simulink model "PMSM_continous"  (R2019b)
settings: Solver=VariableStepAuto  StartTime=0.0  StopTime=2  FixedStep=1/200000  RelTol=1e-3
model workspace (MAT data in the model file):
  K1 = 5
  K2 = 2000
  Kr = 5
  Ld = 0.01024
  Lq = 0.01024
  P = 10
  Rs = 0.732
  Ts = 5e-05
  Tsim = 5e-05
  Tsim1 = 5e-07
  Udc = 150
  flux = 0.1385
  sigmoid = 0.05
  switch_time = 0.15
undefined symbols (not defined in the file): DiscIntNeverNeededParam, LowerLimit, UpperLimit
libraries: powerlib x9, dspstat3 x4, powerlib_meascontrol x4, simulink x4, fuzblock x4, eeTransforms x2, powerlib_extras x1
settings Model: SimulationMode=accelerator  Creator=Downstream  LastModifiedBy=97252
settings SolverCC: ZeroCrossAlgorithm=Adaptive  AlgebraicLoopSolver=LineSearch
settings DataIOCC: ReturnWorkspaceOutputs=off
settings OptimizationCC: DefaultUnderspecifiedDataType=single  EfficientMapNaN2IntZero=off
settings DebuggingCC: IgnoredZcDiagnostic=none  ArithmeticOperatorsInVariantConditions=warning
settings HardwareCC: TargetBitPerPointer=64  TargetBitPerSizeT=64  TargetBitPerPtrDiffT=64  TargetLongLongMode=on  TargetIntDivRoundTo=Zero  TargetEndianess=LittleEndian  TargetWordSize=64  TargetHWDeviceType=MATLAB Host  ProdEqTarget=off
settings SFSimCC: CustomCodeUndefinedFunction=UseInterfaceOnly
settings CodeAppCC: MaxIdLength=128
settings GRTTargetCC: TargetLangStandard=C89/C90 (ANSI)  CombineOutputUpdateFcns=off  GRTInterface=on

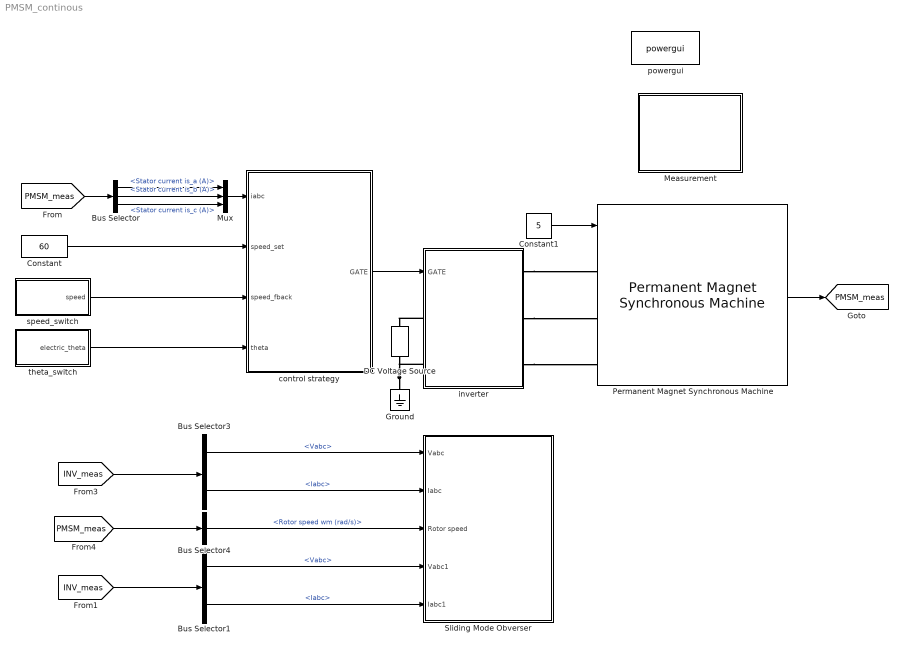
== system PMSM_continous ==
  Bus Selector : BusSelector  OutputSignals=Stator current is_a (A),Stator current is_b (A),Stator current is_c (A)
  Bus Selector1 : BusSelector  OutputSignals=Vabc,Iabc
  Bus Selector3 : BusSelector  OutputSignals=Vabc,Iabc
  Bus Selector4 : BusSelector  OutputSignals=Rotor speed wm (rad/s)
  Constant : Constant  Value=60
  Constant1 : Constant  Value=5
  DC Voltage Source : powerlib/Electrical Sources/DC Voltage Source  Amplitude=Udc  Measurements=None
      settings: SourceProductName=Simscape Electrical
  Ground : powerlib/Elements/Ground  LConnTagsString=a
      settings: SourceProductName=Simscape Electrical
  "Measurement " : Subsystem
  Mux : Mux  Inputs=3
  Permanent Magnet Synchronous Machine : powerlib/Machines/Permanent Magnet Synchronous Machine  NbPhases=3  FluxDistribution=Sinusoidal  RotorType=Salient-pole  MechanicalLoad=Torque Tm  PresetModel=No  ShowDetailedParameters=on  MeasurementBus=off  Resistance=Rs  Inductance=8.5e-3  dqInductances=[Ld, Lq]  La=Ls  MachineConstant=Flux linkage established by magnets (V.s)  Flux=flux  VoltageCst=251.2112  TorqueCst=2.0775  Flat=120  Mechanical=[0.027 0 10 0]  PolePairs=4  InitialConditions=[0,0, 0,0]  InitialConditions5ph=[0 0 0 0 0 0]  RefAngle=Aligned with phase A axis (original Park)  IterativeDiscreteModel=Trapezoidal non iterative  TsBlock=-1  TsPowergui=0
  Sliding Mode Obverser : Subsystem
  control strategy : Subsystem
  "inverter " : Subsystem
  powergui : powerlib/powergui  Priority=1  SimulationMode=Discrete  SampleTime=1/2000000  frequency=60  Iterations=50  frequencyindice=0  Pbase=100e6  ErrMax=1e-4  UnitsV=kV  UnitsW=MW  buscounter=0  FunctionMessages=on  echomessages=on  EnableUseOfTLC=off  CurrentSourceSwitches=off  DisableSnubberDevices=off  DisableRonSwitches=off  DisableVfSwitches=off  DisplayEquations=off  AutomaticDiscreteSolvers=off  SolverType=Tustin/Backward Euler (TBE)  Interpol=off  ExternalGateDelay=off  methode=off  Ts=100  x0status=blocks  SPID=off  SwTol=0  HookPort=off  NonlinearTolerance=1e-4  nMaxIteration=100  ContinueOnMaxIteration=off  RestoreLinks=warning  ResistiveCurrentMeasurement=off  Frange=[0:2:500]  Ylog=off  Xlog=on  ShowGrid=off  save=off  variable=ZData  structure=0  ZoomFFT=off  StartTime=0.0  cycles=1  DisplayStyle=1  fundamental=60  FreqAxis=off  MaxFrequency=1000  frequencyindicesteady=1  RmsSteady=1  display=off
      settings: SourceProductName=Simscape Electrical
  speed_switch : Subsystem
  theta_switch : Subsystem
  tag scope: PMSM_meas=global
  wires:
  Permanent Magnet Synchronous Machine/1 -> [PMSM_meas]
  control strategy/1(GATE) -> "inverter "/1("GATE ")
  [PMSM_meas] -> Bus Selector/1
  Bus Selector/1 -> Mux/1  "<Stator current is_a (A)>"
  Bus Selector/2 -> Mux/2  "<Stator current is_b (A)>"
  Bus Selector/3 -> Mux/3  "<Stator current is_c (A)>"
  Mux/1 -> control strategy/1(iabc)
  Constant1/1 -> Permanent Magnet Synchronous Machine/1
  [PMSM_meas] -> Bus Selector4/1
  Bus Selector4/1 -> Sliding Mode Obverser/3(Rotor speed)  "<Rotor speed wm (rad/s)>"
  Bus Selector3/1 -> Sliding Mode Obverser/1(Vabc)  "<Vabc>"
  Bus Selector3/2 -> Sliding Mode Obverser/2(Iabc)  "<Iabc>"
  [INV_meas] -> Bus Selector3/1
  theta_switch/1(electric_theta) -> control strategy/4(theta)
  speed_switch/1(speed) -> control strategy/3(speed_fback)
  [INV_meas] -> Bus Selector1/1
  Bus Selector1/1 -> Sliding Mode Obverser/4(Vabc1)  "<Vabc>"
  Bus Selector1/2 -> Sliding Mode Obverser/5(Iabc1)  "<Iabc>"
  Constant/1 -> control strategy/2(speed_set)
  connections:
  Ground/LConn1 -- "inverter "/LConn2 -- DC Voltage Source/LConn1
  "inverter "/LConn1 -- DC Voltage Source/RConn1
  "inverter "/RConn1 -- Permanent Magnet Synchronous Machine/LConn1
  "inverter "/RConn2 -- Permanent Magnet Synchronous Machine/LConn2
  "inverter "/RConn3 -- Permanent Magnet Synchronous Machine/LConn3

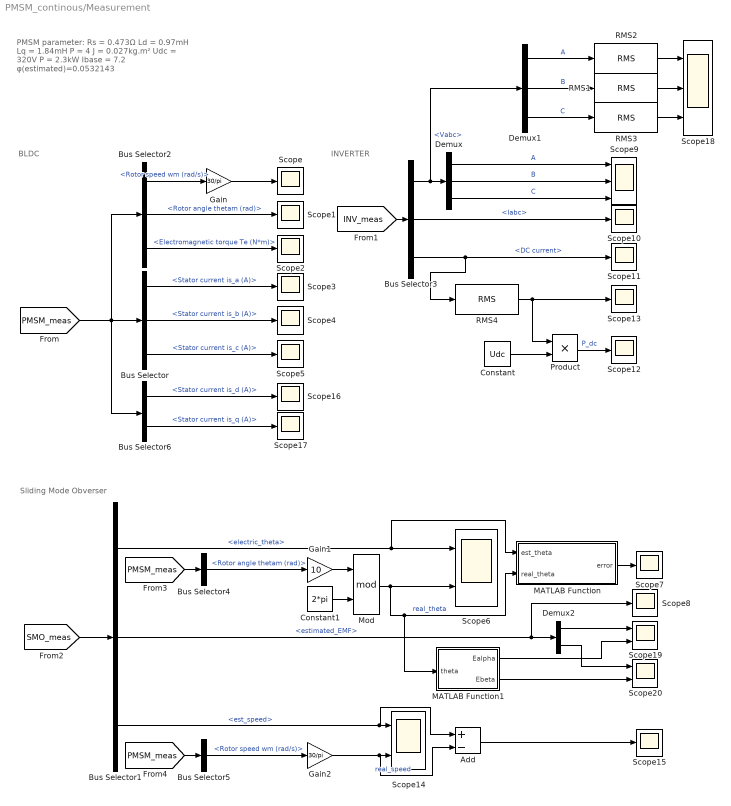
== system PMSM_continous/Measurement  ==
  note: Sliding Mode Obverser
  note: INVERTER
  note: BLDC
  note: PMSM parameter:
      | Rs = 0.473Ω
      | Ld = 0.97mH
      | Lq = 1.84mH
      | P  = 4
      | J   = 0.027kg.m²
      | Udc = 320V
      | P   = 2.3kW
      | Ibase  = 7.2
      | φ(estimated)=0.0532143
  Add : Sum  Inputs=+-
  Bus Selector : BusSelector  OutputSignals=Stator current is_a (A),Stator current is_b (A),Stator current is_c (A)
  Bus Selector1 : BusSelector  OutputSignals=electric_theta,estimated_EMF,est_speed
  Bus Selector2 : BusSelector  OutputSignals=Rotor speed wm (rad/s),Rotor angle thetam (rad),Electromagnetic torque Te (N*m)
  Bus Selector3 : BusSelector  OutputSignals=Vabc,Iabc,DC current
  Bus Selector4 : BusSelector  OutputSignals=Rotor angle thetam (rad)
  Bus Selector5 : BusSelector  OutputSignals=Rotor speed wm (rad/s)
  Bus Selector6 : BusSelector  OutputSignals=Stator current is_d (A),Stator current is_q (A)
  Constant : Constant  Value=Udc
  Constant1 : Constant  Value=2*pi
  Demux : Demux  Outputs=3
  Demux1 : Demux  Outputs=3
  Demux2 : Demux  Outputs=2
  Gain : Gain  Gain=30/pi
  Gain1 : Gain  Gain=10
  Gain2 : Gain  Gain=30/pi
  MATLAB Function : MATLAB Function  TreatAsAtomicUnit=on
  MATLAB Function1 : MATLAB Function  TreatAsAtomicUnit=on
  Mod : Math  Operator=mod  SaturateOnIntegerOverflow=on
  Product : Product
  RMS{1..4} (4 alike) : dspstat3/RMS  run=on  directionMode=Each column  dimension=1  reset_popup=None
  Scope{,1..5,7..8,10..13,15..17} (15 alike) : Scope
  Scope{6,14,19..20} (4 alike) : Scope  NumInputPorts=2
  Scope18 : Scope  NumInputPorts=3
  Scope9 : Scope  NumInputPorts=3
  wires:
  [PMSM_meas] -> Bus Selector6/1, Bus Selector2/1, Bus Selector/1
  Bus Selector2/1 -> Gain/1  "<Rotor speed wm (rad/s)>"
  Bus Selector2/2 -> Scope1/1  "<Rotor angle thetam (rad)>"
  Bus Selector2/3 -> Scope2/1  "<Electromagnetic torque Te (N*m)>"
  Bus Selector/1 -> Scope3/1  "<Stator current is_a (A)>"
  Bus Selector/2 -> Scope4/1  "<Stator current is_b (A)>"
  Bus Selector/3 -> Scope5/1  "<Stator current is_c (A)>"
  [INV_meas] -> Bus Selector3/1
  Bus Selector3/1 -> Demux1/1, Demux/1  "<Vabc>"
  Bus Selector3/2 -> Scope10/1  "<Iabc>"
  Gain/1 -> Scope/1
  Bus Selector3/3 -> RMS4/1, Scope11/1  "<DC current>"
  Constant/1 -> Product/2
  Product/1 -> Scope12/1  "P_dc"
  Demux/2 -> Scope9/2  "B"
  Demux/1 -> Scope9/1  "A"
  Demux/3 -> Scope9/3  "C"
  RMS4/1 -> Product/1, Scope13/1
  [SMO_meas] -> Bus Selector1/1
  Bus Selector1/1 -> MATLAB Function/1(est_theta), Scope6/1  "<electric_theta>"
  Constant1/1 -> Mod/2
  Gain1/1 -> Mod/1
  Bus Selector4/1 -> Gain1/1  "<Rotor angle thetam (rad)>"
  [PMSM_meas] -> Bus Selector4/1
  Mod/1 -> MATLAB Function1/1(theta), MATLAB Function/2(real_theta), Scope6/2  "real_theta"
  MATLAB Function/1(error) -> Scope7/1
  Bus Selector1/3 -> Add/1, Scope14/1  "<est_speed>"
  [PMSM_meas] -> Bus Selector5/1
  Bus Selector5/1 -> Gain2/1  "<Rotor speed wm (rad/s)>"
  Gain2/1 -> Add/2, Scope14/2  "real_speed"
  Add/1 -> Scope15/1
  Bus Selector6/1 -> Scope16/1  "<Stator current is_d (A)>"
  Bus Selector6/2 -> Scope17/1  "<Stator current is_q (A)>"
  Demux1/1 -> RMS2/1  "A"
  Demux1/2 -> RMS1/1  "B"
  Demux1/3 -> RMS3/1  "C"
  RMS2/1 -> Scope18/1
  RMS1/1 -> Scope18/2
  RMS3/1 -> Scope18/3
  Bus Selector1/2 -> Scope8/1, Demux2/1  "<estimated_EMF>"
  Demux2/1 -> Scope19/1
  MATLAB Function1/1(Ealpha) -> Scope19/2
  MATLAB Function1/2(Ebeta) -> Scope20/2
  Demux2/2 -> Scope20/1

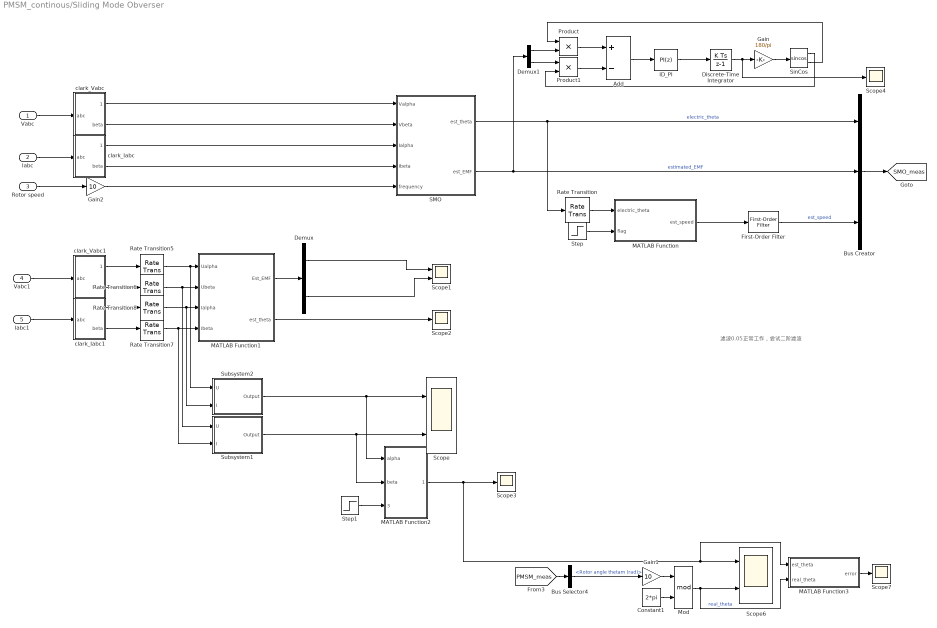
== system PMSM_continous/Sliding Mode Obverser ==
  note: 滤波0.05正常工作，尝试二阶滤波
  Vabc : Inport
  Iabc : Inport  Port=2
  Rotor speed : Inport  Port=3
  Vabc1 : Inport  Port=4
  Iabc1 : Inport  Port=5
  Add : Sum  Inputs=+-
  Bus Creator : BusCreator  Inputs=3
  Bus Selector4 : BusSelector  OutputSignals=Rotor angle thetam (rad)
  Constant1 : Constant  Value=2*pi
  Demux : Demux  Outputs=2
  Demux1 : Demux  Outputs=2
  Discrete-Time Integrator : DiscreteIntegrator  SampleTime=-1  ICPrevOutput=DiscIntNeverNeededParam  ICPrevScaledInput=DiscIntNeverNeededParam
  First-Order Filter : powerlib_meascontrol/Filters/First-Order Filter  FilterType=Lowpass  Tc=1/100  Ts=1/20000  Initialize=off  Vac_Init=[0, 0, 60]  Vdc_Init=0  PlotResponse=off  FreqRange="[0,  200,  1]"
      settings: SourceProductName=Simscape Electrical
  Gain : Gain  Gain=180/pi
  Gain1 : Gain  Gain=10
  Gain2 : Gain  Gain=10
  "ID_PI " : simulink/Continuous/PID Controller  Controller=PI  Form=Parallel  TimeDomain=Discrete-time  SampleTime=-1  IntegratorMethod=Forward Euler  FilterMethod=Forward Euler  ControllerParametersSource=internal  P=300  I=1  D=0  UseFilter=on  N=100  TunerSelectOption=Transfer Function Based (PID Tuner App)  InitialConditionSource=internal  InitialConditionForIntegrator=0  InitialConditionForFilter=0  DifferentiatorICPrevScaledInput=0  ExternalReset=none  TrackingMode=off  Kt=1  LimitOutput=on  UpperSaturationLimit=sqrt(3)/2  LowerSaturationLimit=-sqrt(3)/2  LinearizeAsGain=on  AntiWindupMode=none  Kb=1  POutMin=[]  POutMax=[]  IOutMin=[]  IOutMax=[]  DOutMin=[]  DOutMax=[]  NOutMin=[]  NOutMax=[]  SumOutMin=[]  SumOutMax=[]  SaturationOutMin=[]  SaturationOutMax=[]  PParamMin=[]  PParamMax=[]  IParamMin=[]  IParamMax=[]  DParamMin=[]  DParamMax=[]  NParamMin=[]  NParamMax=[]  KbParamMin=[]  KbParamMax=[]  KtParamMin=[]  KtParamMax=[]  KbOutMin=[]  KbOutMax=[]  KtOutMin=[]  KtOutMax=[]  IntegratorOutMin=[]  IntegratorOutMax=[]  FilterOutMin=[]  FilterOutMax=[]  SumI1OutMin=[]  SumI1OutMax=[]  SumI2OutMin=[]  SumI2OutMax=[]  SumI3OutMin=[]  SumI3OutMax=[]  SumI4OutMin=[]  SumI4OutMax=[]  SumDOutMin=[]  SumDOutMax=[]  DifferentiatorOutMin=[]  DifferentiatorOutMax=[]  FilterDiffOutCoefMin=[]  FilterDiffOutCoefMax=[]  ReciprocalOutMin=[]  ReciprocalOutMax=[]  SumDenOutMin=[]  SumDenOutMax=[]  SumNumOutMin=[]  SumNumOutMax=[]  DivideOutMin=[]  DivideOutMax=[]  IntegratorContinuousStateAttributes=''  IntegratorStateMustResolveToSignalObject=off  IntegratorRTWStateStorageClass=Auto  FilterContinuousStateAttributes=''  FilterStateMustResolveToSignalObject=off  FilterRTWStateStorageClass=Auto  ParallelPVariant=InternalParameters  IdealPVariant=Disabled  IVariant=InternalParameters  DVariant=Disabled  IntegratorVariant=Discrete  SatVariant=Enabled  AWVariant=Passthrough  PCopyVariant=Disabled  TRVariant=Disabled  FdbkBlocksVariant=Forward  IdealPFdbkVariant=Disabled  SatFdbkVariant=Disabled  DerivativeFilterVariant=Disabled  NVariant=Disabled  NCopyVariant=Disabled_SignalSpec  FilterICVariant=Disabled  IntegratorICVariant=InternalICs  ExternalResetVariant=Disabled  TRSumVariant=Passthrough  SumFdbkVariant=Disabled  SumVariant=Sum_PI
  MATLAB Function : MATLAB Function  TreatAsAtomicUnit=on
  MATLAB Function1 : MATLAB Function  TreatAsAtomicUnit=on
  MATLAB Function2 : MATLAB Function  TreatAsAtomicUnit=on
  MATLAB Function3 : MATLAB Function  TreatAsAtomicUnit=on
  Mod : Math  Operator=mod  SaturateOnIntegerOverflow=on
  Product : Product
  Product1 : Product
  Rate Transition : RateTransition  OutPortSampleTime=Ts
  Rate Transition{5..8} (4 alike) : RateTransition  OutPortSampleTime=Tsim
  SMO : MATLAB Function  TreatAsAtomicUnit=on
  Scope : Scope  NumInputPorts=2
  Scope1 : Scope  NumInputPorts=2
  Scope{2..4,7} (4 alike) : Scope
  Scope6 : Scope  NumInputPorts=2
  SinCos : Trigonometry  Operator=sincos
  Step : Step  Time=switch_time/2  SampleTime=Ts
  Step1 : Step  Time=0  After=0  SampleTime=0
  Subsystem1 : Subsystem
  Subsystem2 : Subsystem
  clark_Iabc : Subsystem
  clark_Iabc1 : Subsystem
  clark_Vabc : Subsystem
  clark_Vabc1 : Subsystem
  tag scope: SMO_meas=global
  wires:
  Rate Transition/1 -> MATLAB Function/1(electric_theta)
  MATLAB Function/1(est_speed) -> First-Order Filter/1
  Step/1 -> MATLAB Function/2(flag)
  First-Order Filter/1 -> Bus Creator/3  "est_speed"
  Bus Creator/1 -> [SMO_meas]
  SMO/2(est_EMF) -> Bus Creator/2, Demux1/1  "estimated_EMF"
  SMO/1(est_theta) -> Rate Transition/1, Bus Creator/1  "electric_theta"
  Vabc/1 -> clark_Vabc/1(abc)
  Iabc/1 -> clark_Iabc/1(abc)
  Rotor speed/1 -> Gain2/1
  clark_Vabc1/1(alpha) -> Rate Transition5/1
  clark_Vabc1/2(beta) -> Rate Transition6/1
  clark_Iabc1/1(alpha) -> Rate Transition8/1
  clark_Iabc1/2(beta) -> Rate Transition7/1
  MATLAB Function1/1(Est_EMF) -> Demux/1
  Demux/1 -> Scope1/1
  Demux/2 -> Scope1/2
  MATLAB Function1/2(est_theta) -> Scope2/1
  Iabc1/1 -> clark_Iabc1/1(abc)
  Vabc1/1 -> clark_Vabc1/1(abc)
  [PMSM_meas] -> Bus Selector4/1
  Bus Selector4/1 -> Gain1/1  "<Rotor angle thetam (rad)>"
  Mod/1 -> Scope6/2, MATLAB Function3/2(real_theta)  "real_theta"
  MATLAB Function3/1(error) -> Scope7/1
  Gain1/1 -> Mod/1
  MATLAB Function2/1(Est_theta) -> Scope3/1, MATLAB Function3/1(est_theta), Scope6/1
  Constant1/1 -> Mod/2
  Subsystem2/1(Output) -> Scope/1, MATLAB Function2/1(alpha)
  Subsystem1/1(Output) -> MATLAB Function2/2(beta), Scope/2
  Step1/1 -> MATLAB Function2/3(compansite)
  Rate Transition5/1 -> Subsystem2/1(U), MATLAB Function1/1(Ualpha)
  Rate Transition6/1 -> Subsystem1/1(U), MATLAB Function1/2(Ubeta)
  Rate Transition7/1 -> Subsystem1/2(I), MATLAB Function1/4(Ibeta)
  Rate Transition8/1 -> Subsystem2/2(I), MATLAB Function1/3(Ialpha)
  clark_Iabc/1(alpha) -> SMO/3(Ialpha)
  clark_Vabc/1(alpha) -> SMO/1(Valpha)
  clark_Vabc/2(beta) -> SMO/2(Vbeta)
  clark_Iabc/2(beta) -> SMO/4(Ibeta)
  Gain2/1 -> SMO/5(frequency)
  Demux1/1 -> Product/2
  Demux1/2 -> Product1/1
  Product/1 -> Add/1
  Product1/1 -> Add/2
  Add/1 -> "ID_PI "/1
  "ID_PI "/1 -> Discrete-Time Integrator/1
  Discrete-Time Integrator/1 -> Gain/1, Scope4/1
  SinCos/2 -> Product/1
  SinCos/1 -> Product1/2
  Gain/1 -> SinCos/1

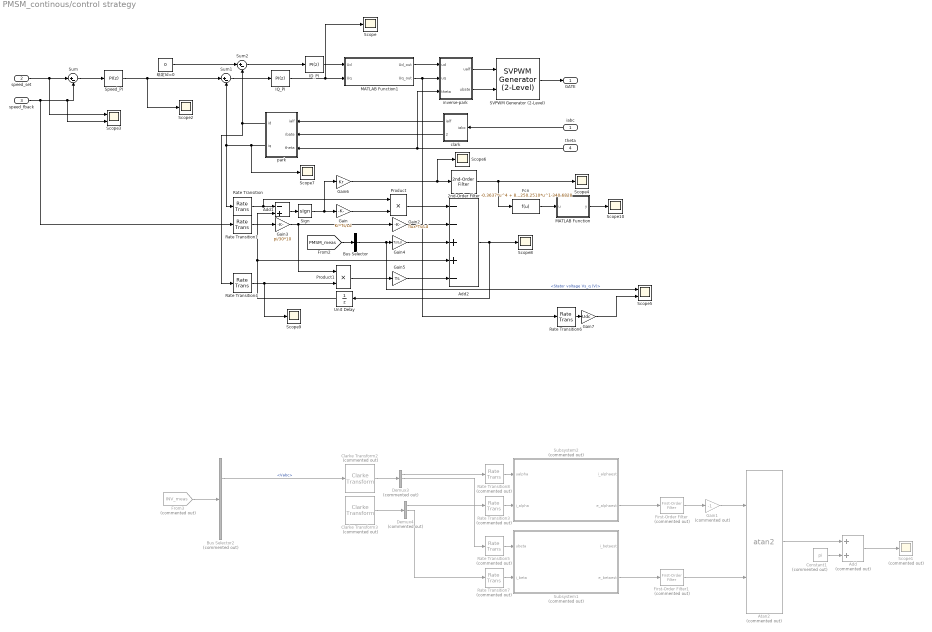
== system PMSM_continous/control strategy ==
  iabc : Inport
  speed_set : Inport  Port=2
  speed_fback : Inport  Port=3
  theta : Inport  Port=4
  2nd-Order Filter : powerlib_extras/Control  Blocks/2nd-Order Filter  FilterType=Lowpass  Fo=50  Zeta=0.707  Initialize=off  Vac_Init=[1 45 60]  Vdc_Init=-0.5  PlotResponse=off  param1=[1 500 1]
      settings: SourceProductName=Simscape Electrical  SourceProductBaseCode=PS
  Add : Sum  Commented=on
  Add1 : Sum  Inputs=-+
  Add2 : Sum  Inputs=--++-
  Atan2 : Trigonometry  Commented=on  Operator=atan2
  Bus Selector : BusSelector  OutputSignals=Stator voltage Vs_q (V)
  Bus Selector2 : BusSelector  Commented=on  OutputSignals=Vabc,Iabc
  Clarke Transform2 : eeTransforms/Clarke Transform  Commented=on  PowerInvariant=off
      settings: SourceProductName=Simscape Electrical  SourceProductBaseCode=PS
  Clarke Transform3 : eeTransforms/Clarke Transform  Commented=on  PowerInvariant=off
      settings: SourceProductName=Simscape Electrical  SourceProductBaseCode=PS
  Constant1 : Constant  Commented=on  Value=pi
  Demux3 : Demux  Commented=on  Outputs=3
  Demux4 : Demux  Commented=on  Outputs=3
  Fcn : Fcn  Expr=-0.3637*u^4 + 8.1652*u^3 - 68.0962*u^2 +250.2510*u^1-340.6828
  First-Order Filter : powerlib_meascontrol/Filters/First-Order Filter  Commented=on  FilterType=Lowpass  Tc=150*pi/30*8*Ts*5  Ts=0  Initialize=off  Vac_Init=[0, 0, 60]  Vdc_Init=0  PlotResponse=off  FreqRange="[0,  200,  1]"
      settings: SourceProductName=Simscape Electrical
  First-Order Filter1 : powerlib_meascontrol/Filters/First-Order Filter  Commented=on  FilterType=Lowpass  Tc=150*pi/30*8*Ts*5  Ts=0  Initialize=off  Vac_Init=[0, 0, 60]  Vdc_Init=0  PlotResponse=off  FreqRange="[0,  200,  1]"
      settings: SourceProductName=Simscape Electrical
  From3 : From  Commented=on  GotoTag=INV_meas  TagVisibility=global
  Gain : Gain  Gain=Kr*Ts/Ld
  Gain1 : Gain  Commented=on  Gain=-1
  Gain2 : Gain  Gain=flux*Ts/Ld
  Gain3 : Gain  Gain=pi/30*10
  Gain4 : Gain  Gain=Ts/Ld
  Gain5 : Gain  Gain=Ts
  Gain6 : Gain  Gain=Kr
  Gain7 : Gain  Gain=Udc
  "ID_PI " : simulink/Continuous/PID Controller  Controller=PI  Form=Parallel  TimeDomain=Discrete-time  SampleTime=Ts  IntegratorMethod=Forward Euler  FilterMethod=Forward Euler  ControllerParametersSource=internal  P=1500*Ld/Udc  I=1500*Rs/Udc  D=0  UseFilter=on  N=100  TunerSelectOption=Transfer Function Based (PID Tuner App)  InitialConditionSource=internal  InitialConditionForIntegrator=0  InitialConditionForFilter=0  DifferentiatorICPrevScaledInput=0  ExternalReset=none  TrackingMode=off  Kt=1  LimitOutput=on  UpperSaturationLimit=sqrt(3)/2  LowerSaturationLimit=-sqrt(3)/2  LinearizeAsGain=on  AntiWindupMode=none  Kb=1  POutMin=[]  POutMax=[]  IOutMin=[]  IOutMax=[]  DOutMin=[]  DOutMax=[]  NOutMin=[]  NOutMax=[]  SumOutMin=[]  SumOutMax=[]  SaturationOutMin=[]  SaturationOutMax=[]  PParamMin=[]  PParamMax=[]  IParamMin=[]  IParamMax=[]  DParamMin=[]  DParamMax=[]  NParamMin=[]  NParamMax=[]  KbParamMin=[]  KbParamMax=[]  KtParamMin=[]  KtParamMax=[]  KbOutMin=[]  KbOutMax=[]  KtOutMin=[]  KtOutMax=[]  IntegratorOutMin=[]  IntegratorOutMax=[]  FilterOutMin=[]  FilterOutMax=[]  SumI1OutMin=[]  SumI1OutMax=[]  SumI2OutMin=[]  SumI2OutMax=[]  SumI3OutMin=[]  SumI3OutMax=[]  SumI4OutMin=[]  SumI4OutMax=[]  SumDOutMin=[]  SumDOutMax=[]  DifferentiatorOutMin=[]  DifferentiatorOutMax=[]  FilterDiffOutCoefMin=[]  FilterDiffOutCoefMax=[]  ReciprocalOutMin=[]  ReciprocalOutMax=[]  SumDenOutMin=[]  SumDenOutMax=[]  SumNumOutMin=[]  SumNumOutMax=[]  DivideOutMin=[]  DivideOutMax=[]  IntegratorContinuousStateAttributes=''  IntegratorStateMustResolveToSignalObject=off  IntegratorRTWStateStorageClass=Auto  FilterContinuousStateAttributes=''  FilterStateMustResolveToSignalObject=off  FilterRTWStateStorageClass=Auto  ParallelPVariant=InternalParameters  IdealPVariant=Disabled  IVariant=InternalParameters  DVariant=Disabled  IntegratorVariant=Discrete  SatVariant=Enabled  AWVariant=Passthrough  PCopyVariant=Disabled  TRVariant=Disabled  FdbkBlocksVariant=Forward  IdealPFdbkVariant=Disabled  SatFdbkVariant=Disabled  DerivativeFilterVariant=Disabled  NVariant=Disabled  NCopyVariant=Disabled_SignalSpec  FilterICVariant=Disabled  IntegratorICVariant=InternalICs  ExternalResetVariant=Disabled  TRSumVariant=Passthrough  SumFdbkVariant=Disabled  SumVariant=Sum_PI
  "IQ_PI " : simulink/Continuous/PID Controller  Controller=PI  Form=Parallel  TimeDomain=Discrete-time  SampleTime=Ts  IntegratorMethod=Forward Euler  FilterMethod=Forward Euler  ControllerParametersSource=internal  P=1500*Ld/Udc  I=1500*Rs/Udc  D=0  UseFilter=on  N=100  TunerSelectOption=Transfer Function Based (PID Tuner App)  InitialConditionSource=internal  InitialConditionForIntegrator=0  InitialConditionForFilter=0  DifferentiatorICPrevScaledInput=0  ExternalReset=none  TrackingMode=off  Kt=1  LimitOutput=on  UpperSaturationLimit=sqrt(3)/2  LowerSaturationLimit=-sqrt(3)/2  LinearizeAsGain=on  AntiWindupMode=none  Kb=1  POutMin=[]  POutMax=[]  IOutMin=[]  IOutMax=[]  DOutMin=[]  DOutMax=[]  NOutMin=[]  NOutMax=[]  SumOutMin=[]  SumOutMax=[]  SaturationOutMin=[]  SaturationOutMax=[]  PParamMin=[]  PParamMax=[]  IParamMin=[]  IParamMax=[]  DParamMin=[]  DParamMax=[]  NParamMin=[]  NParamMax=[]  KbParamMin=[]  KbParamMax=[]  KtParamMin=[]  KtParamMax=[]  KbOutMin=[]  KbOutMax=[]  KtOutMin=[]  KtOutMax=[]  IntegratorOutMin=[]  IntegratorOutMax=[]  FilterOutMin=[]  FilterOutMax=[]  SumI1OutMin=[]  SumI1OutMax=[]  SumI2OutMin=[]  SumI2OutMax=[]  SumI3OutMin=[]  SumI3OutMax=[]  SumI4OutMin=[]  SumI4OutMax=[]  SumDOutMin=[]  SumDOutMax=[]  DifferentiatorOutMin=[]  DifferentiatorOutMax=[]  FilterDiffOutCoefMin=[]  FilterDiffOutCoefMax=[]  ReciprocalOutMin=[]  ReciprocalOutMax=[]  SumDenOutMin=[]  SumDenOutMax=[]  SumNumOutMin=[]  SumNumOutMax=[]  DivideOutMin=[]  DivideOutMax=[]  IntegratorContinuousStateAttributes=''  IntegratorStateMustResolveToSignalObject=off  IntegratorRTWStateStorageClass=Auto  FilterContinuousStateAttributes=''  FilterStateMustResolveToSignalObject=off  FilterRTWStateStorageClass=Auto  ParallelPVariant=InternalParameters  IdealPVariant=Disabled  IVariant=InternalParameters  DVariant=Disabled  IntegratorVariant=Discrete  SatVariant=Enabled  AWVariant=Passthrough  PCopyVariant=Disabled  TRVariant=Disabled  FdbkBlocksVariant=Forward  IdealPFdbkVariant=Disabled  SatFdbkVariant=Disabled  DerivativeFilterVariant=Disabled  NVariant=Disabled  NCopyVariant=Disabled_SignalSpec  FilterICVariant=Disabled  IntegratorICVariant=InternalICs  ExternalResetVariant=Disabled  TRSumVariant=Passthrough  SumFdbkVariant=Disabled  SumVariant=Sum_PI
  MATLAB Function : MATLAB Function  TreatAsAtomicUnit=on
  MATLAB Function1 : MATLAB Function  TreatAsAtomicUnit=on
  Product : Product
  Product1 : Product
  Rate Transition{,1,4,6} (4 alike) : RateTransition  OutPortSampleTime=Ts
  Rate Transition3 : RateTransition  Commented=on  OutPortSampleTime=Ts
  Rate Transition5 : RateTransition  Commented=on  OutPortSampleTime=Ts
  Rate Transition7 : RateTransition  Commented=on  OutPortSampleTime=Ts
  Rate Transition8 : RateTransition  Commented=on  InitialCondition=Ts/10  OutPortSampleTime=Ts
  SVPWM Generator (2-Level) : powerlib_meascontrol/Pulse & Signal Generators/SVPWM Generator (2-Level)  InputType=alpha-beta components  SwitchingPattern=Pattern #1  Fc=20e3  ParUref=[0.8 -30 50]  Ts=0
      settings: SourceProductName=Simscape Electrical  SourceProductBaseCode=PS
  Scope{,2,4,6..10} (8 alike) : Scope
  Scope1 : Scope  Commented=on
  Scope3 : Scope  NumInputPorts=2
  Scope5 : Scope  NumInputPorts=2
  Sign : Signum
  Speed_PI : simulink/Continuous/PID Controller  Controller=PI  Form=Parallel  TimeDomain=Discrete-time  SampleTime=Ts*100  IntegratorMethod=Forward Euler  FilterMethod=Forward Euler  ControllerParametersSource=internal  P=0.05  I=1  D=0  UseFilter=on  N=100  TunerSelectOption=Transfer Function Based (PID Tuner App)  InitialConditionSource=internal  InitialConditionForIntegrator=0  InitialConditionForFilter=0  DifferentiatorICPrevScaledInput=0  ExternalReset=none  TrackingMode=off  Kt=1  LimitOutput=on  UpperSaturationLimit=50  LowerSaturationLimit=-50  LinearizeAsGain=on  AntiWindupMode=none  Kb=1  POutMin=[]  POutMax=[]  IOutMin=[]  IOutMax=[]  DOutMin=[]  DOutMax=[]  NOutMin=[]  NOutMax=[]  SumOutMin=[]  SumOutMax=[]  SaturationOutMin=[]  SaturationOutMax=[]  PParamMin=[]  PParamMax=[]  IParamMin=[]  IParamMax=[]  DParamMin=[]  DParamMax=[]  NParamMin=[]  NParamMax=[]  KbParamMin=[]  KbParamMax=[]  KtParamMin=[]  KtParamMax=[]  KbOutMin=[]  KbOutMax=[]  KtOutMin=[]  KtOutMax=[]  IntegratorOutMin=[]  IntegratorOutMax=[]  FilterOutMin=[]  FilterOutMax=[]  SumI1OutMin=[]  SumI1OutMax=[]  SumI2OutMin=[]  SumI2OutMax=[]  SumI3OutMin=[]  SumI3OutMax=[]  SumI4OutMin=[]  SumI4OutMax=[]  SumDOutMin=[]  SumDOutMax=[]  DifferentiatorOutMin=[]  DifferentiatorOutMax=[]  FilterDiffOutCoefMin=[]  FilterDiffOutCoefMax=[]  ReciprocalOutMin=[]  ReciprocalOutMax=[]  SumDenOutMin=[]  SumDenOutMax=[]  SumNumOutMin=[]  SumNumOutMax=[]  DivideOutMin=[]  DivideOutMax=[]  IntegratorContinuousStateAttributes=''  IntegratorStateMustResolveToSignalObject=off  IntegratorRTWStateStorageClass=Auto  FilterContinuousStateAttributes=''  FilterStateMustResolveToSignalObject=off  FilterRTWStateStorageClass=Auto  ParallelPVariant=InternalParameters  IdealPVariant=Disabled  IVariant=InternalParameters  DVariant=Disabled  IntegratorVariant=Discrete  SatVariant=Enabled  AWVariant=Passthrough  PCopyVariant=Disabled  TRVariant=Disabled  FdbkBlocksVariant=Forward  IdealPFdbkVariant=Disabled  SatFdbkVariant=Disabled  DerivativeFilterVariant=Disabled  NVariant=Disabled  NCopyVariant=Disabled_SignalSpec  FilterICVariant=Disabled  IntegratorICVariant=InternalICs  ExternalResetVariant=Disabled  TRSumVariant=Passthrough  SumFdbkVariant=Disabled  SumVariant=Sum_PI
  Subsystem1 : Subsystem  Commented=on
  Subsystem2 : Subsystem  Commented=on
  Sum : Sum  Inputs=|+-
  Sum1 : Sum  Inputs=|+-
  Sum2 : Sum  Inputs=|+-
  Unit Delay : UnitDelay  SampleTime=-1  HasFrameUpgradeWarning=on
  clark : Subsystem
  inverse-park : Subsystem
  park : Subsystem
  给定Id=0 : Constant  Value=0
  GATE : Outport  VectorParamsAs1DForOutWhenUnconnected=off
  wires:
  SVPWM Generator (2-Level)/1 -> GATE/1
  park/2(iq) -> Scope7/1, Sum1/2, Rate Transition/1
  Sum2/1 -> "ID_PI "/1
  Sum1/1 -> "IQ_PI "/1
  park/1("id ") -> Sum2/2, Rate Transition4/1
  clark/1(ialf) -> park/1(ialf)
  clark/2(ibate) -> park/2(ibate)
  给定Id=0/1 -> Sum2/1
  Sum/1 -> Speed_PI/1
  speed_set/1 -> Scope3/1, Sum/1
  inverse-park/2(ubate) -> SVPWM Generator (2-Level)/2
  inverse-park/1("ualf ") -> SVPWM Generator (2-Level)/1
  Subsystem2/2(e_alphaest) -> First-Order Filter/1
  Subsystem1/2(e_betaest) -> First-Order Filter1/1
  First-Order Filter/1 -> Gain1/1
  Gain1/1 -> Atan2/1
  First-Order Filter1/1 -> Atan2/2
  Atan2/1 -> Add/1
  Constant1/1 -> Add/2
  Demux4/2 -> Rate Transition7/1
  From3/1 -> Bus Selector2/1
  Clarke Transform2/1 -> Demux3/1
  Demux3/1 -> Rate Transition8/1
  Clarke Transform3/1 -> Demux4/1
  Demux3/2 -> Rate Transition5/1
  Demux4/1 -> Rate Transition3/1
  Bus Selector2/1 -> Clarke Transform2/1  "<Vabc>"
  Rate Transition8/1 -> Subsystem2/1(ualpha)
  Rate Transition5/1 -> Subsystem1/1(ubeta)
  Rate Transition3/1 -> Subsystem2/2(i_alpha)
  Rate Transition7/1 -> Subsystem1/2(i_beta)
  Add/1 -> Scope1/1
  iabc/1 -> clark/1(iabc)
  theta/1 -> inverse-park/3(theta), park/3(theta)
  "ID_PI "/1 -> MATLAB Function1/1(Ud)
  "IQ_PI "/1 -> Scope/1, MATLAB Function1/2(Uq)
  MATLAB Function1/1(Ud_out) -> inverse-park/1(ud)
  Speed_PI/1 -> Scope2/1, Sum1/1
  Add1/1 -> Sign/1
  Gain2/1 -> Add2/2
  speed_fback/1 -> Rate Transition1/1, Scope3/2, Sum/2
  Gain3/1 -> Product1/1, Gain2/1
  Gain4/1 -> Add2/3
  Add2/1 -> Scope8/1, Unit Delay/1
  Unit Delay/1 -> Add1/2, Add2/4
  2nd-Order Filter/1 -> Fcn/1, Scope4/1
  Rate Transition/1 -> Product/1, Add1/1
  Rate Transition1/1 -> Gain3/1
  Gain/1 -> Product/2
  Product/1 -> Add2/1
  Rate Transition4/1 -> Product1/2, Scope9/1
  Product1/1 -> Gain5/1
  Gain5/1 -> Add2/5
  Sign/1 -> Gain6/1, Gain/1
  Fcn/1 -> MATLAB Function/1(u)
  MATLAB Function/1(y) -> Scope10/1
  Gain6/1 -> Scope6/1, 2nd-Order Filter/1
  MATLAB Function1/2(Uq_out) -> Rate Transition6/1, inverse-park/2(uq)
  [PMSM_meas] -> Bus Selector/1
  Bus Selector/1 -> Scope5/1, Gain4/1  "<Stator voltage Vs_q (V)>"
  Rate Transition6/1 -> Gain7/1
  Gain7/1 -> Scope5/2

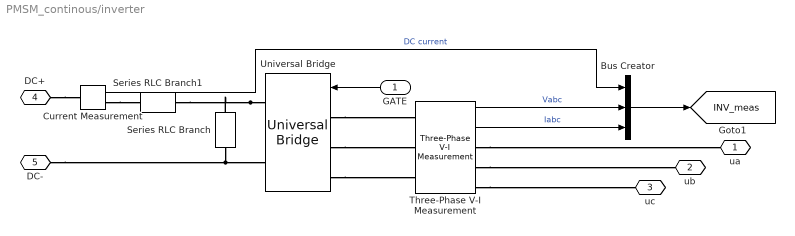
== system PMSM_continous/inverter  ==
  "GATE " : Inport
  Bus Creator : BusCreator  Inputs=3
  Current Measurement : powerlib/Measurements/Current Measurement  PhasorSimulation=off  OutputType=Complex  PSBequivalent=0
      settings: SourceProductName=Simscape Electrical
  Series RLC Branch : powerlib/Elements/Series RLC Branch  LConnTagsString=__new0  RConnTagsString=__new0  BranchType=C  Resistance=1  Inductance=1e-3  SetiL0=off  InitialCurrent=0  Capacitance=5e-3  Setx0=on  InitialVoltage=Udc  Measurements=None
      settings: SourceProductName=Simscape Electrical
  Series RLC Branch1 : powerlib/Elements/Series RLC Branch  LConnTagsString=__new0  RConnTagsString=__new0  BranchType=R  Resistance=0.001  Inductance=1e-3  SetiL0=off  InitialCurrent=0  Capacitance=50e-6  Setx0=off  InitialVoltage=0  Measurements=None
      settings: SourceProductName=Simscape Electrical
  Three-Phase V-I Measurement : powerlib/Measurements/Three-Phase V-I Measurement  VoltageMeasurement=phase-to-ground  SetLabelV=off  LabelV=Vabc  Vpu=off  VpuLL=off  CurrentMeasurement=yes  SetLabelI=off  LabelI=Iabc  Ipu=off  Pbase=100e6  Vbase=500e3  OutputType=Complex  PhasorSimulation=off  PSBequivalent=0
      settings: SourceProductName=Simscape Electrical
  Universal Bridge : powerlib/Power Electronics/Universal Bridge  Arms=3  SnubberResistance=1e5  SnubberCapacitance=inf  Device=IGBT / Diodes  Ron=1e-3  Lon=0  ForwardVoltages="[  0  0  ]"  ForwardVoltage=0  GTOparameters=[ 10e-6 , 20e-6 ]  IGBTparameters=[ 1e-6 , 2e-6 ]  Measurements=None  Measurements_2=None  converterType=Rectifier
      settings: SourceProductName=Simscape Electrical
  ua : PMIOPort  Side=Right
  ub : PMIOPort  Port=2  Side=Right
  uc : PMIOPort  Port=3  Side=Right
  DC+ : PMIOPort  Port=4  Side=Left
  DC- : PMIOPort  Port=5  Side=Left
  tag scope: INV_meas=global
  wires:
  "GATE "/1 -> Universal Bridge/1
  Three-Phase V-I Measurement/1 -> Bus Creator/2  "Vabc"
  Bus Creator/1 -> [INV_meas]
  Three-Phase V-I Measurement/2 -> Bus Creator/3  "Iabc"
  Current Measurement/1 -> Bus Creator/1  "DC current"
  connections:
  Universal Bridge/LConn1 -- Three-Phase V-I Measurement/LConn1
  Universal Bridge/LConn2 -- Three-Phase V-I Measurement/LConn2
  DC-/RConn1 -- Series RLC Branch/RConn1 -- Universal Bridge/RConn2
  Universal Bridge/LConn3 -- Three-Phase V-I Measurement/LConn3
  Three-Phase V-I Measurement/RConn1 -- ua/RConn1
  Three-Phase V-I Measurement/RConn2 -- ub/RConn1
  Three-Phase V-I Measurement/RConn3 -- uc/RConn1
  Universal Bridge/RConn1 -- Series RLC Branch1/RConn1 -- Series RLC Branch/LConn1
  DC+/RConn1 -- Current Measurement/LConn1
  Current Measurement/RConn1 -- Series RLC Branch1/LConn1

== system PMSM_continous/speed_switch ==
  Bus Selector4 : BusSelector  OutputSignals=Rotor speed wm (rad/s)
  Gain : Gain  Gain=30/pi
  speed : Outport  VectorParamsAs1DForOutWhenUnconnected=off
  wires:
  [PMSM_meas] -> Bus Selector4/1
  Bus Selector4/1 -> Gain/1  "<Rotor speed wm (rad/s)>"
  Gain/1 -> speed/1

== system PMSM_continous/theta_switch ==
  Bus Selector4 : BusSelector  OutputSignals=Rotor angle thetam (rad)
  Constant1 : Constant  Value=2*pi
  Gain1 : Gain  Gain=10
  Mod : Math  Operator=mod  SaturateOnIntegerOverflow=on
  electric_theta : Outport  VectorParamsAs1DForOutWhenUnconnected=off
  wires:
  [PMSM_meas] -> Bus Selector4/1
  Bus Selector4/1 -> Gain1/1  "<Rotor angle thetam (rad)>"
  Gain1/1 -> Mod/1
  Constant1/1 -> Mod/2
  Mod/1 -> electric_theta/1  "real_theta"

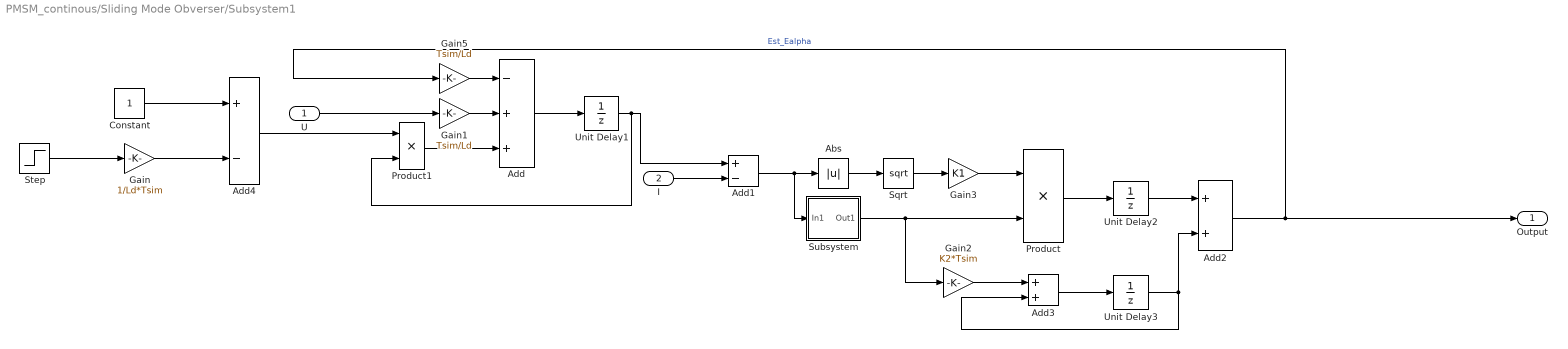
== system PMSM_continous/Sliding Mode Obverser/Subsystem1 ==
  U : Inport
  I : Inport  Port=2
  Abs : Abs
  Add : Sum  Inputs=-++
  Add1 : Sum  Inputs=+-
  Add2 : Sum
  Add3 : Sum
  Add4 : Sum  Inputs=+-
  Constant : Constant  SampleTime=Tsim
  Gain : Gain  Gain=1/Ld*Tsim
  Gain1 : Gain  Gain=Tsim/Ld
  Gain2 : Gain  Gain=K2*Tsim
  Gain3 : Gain  Gain=K1
  Gain5 : Gain  Gain=Tsim/Ld
  Product : Product
  Product1 : Product
  Sqrt : Sqrt  SaturateOnIntegerOverflow=on
  Step : Step  Time=3  Before=0.732  After=0.732+1.3  SampleTime=Tsim
  Subsystem : Subsystem
  Unit Delay1 : UnitDelay  SampleTime=-1  HasFrameUpgradeWarning=on
  Unit Delay2 : UnitDelay  SampleTime=-1  HasFrameUpgradeWarning=on
  Unit Delay3 : UnitDelay  SampleTime=-1  HasFrameUpgradeWarning=on
  Output : Outport
  wires:
  Gain/1 -> Add4/2
  Step/1 -> Gain/1
  Constant/1 -> Add4/1
  Add4/1 -> Product1/1
  Unit Delay3/1 -> Add2/2, Add3/2
  Unit Delay2/1 -> Add2/1
  Unit Delay1/1 -> Product1/2, Add1/1
  Abs/1 -> Sqrt/1
  Add1/1 -> Subsystem/1(In1), Abs/1
  I/1 -> Add1/2
  U/1 -> Gain1/1
  Sqrt/1 -> Gain3/1
  Gain3/1 -> Product/1
  Product1/1 -> Add/3
  Add2/1 -> Gain5/1, Output/1  "Est_Ealpha"
  Gain1/1 -> Add/2
  Subsystem/1(Out1) -> Product/2, Gain2/1
  Product/1 -> Unit Delay2/1
  Gain5/1 -> Add/1
  Add/1 -> Unit Delay1/1
  Add3/1 -> Unit Delay3/1
  Gain2/1 -> Add3/1

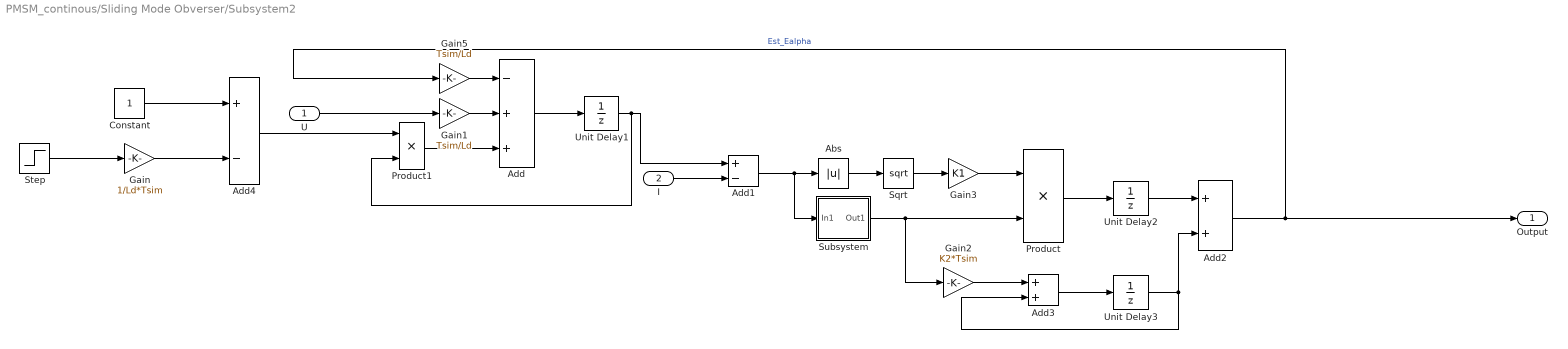
== system PMSM_continous/Sliding Mode Obverser/Subsystem2 ==
  U : Inport
  I : Inport  Port=2
  Abs : Abs
  Add : Sum  Inputs=-++
  Add1 : Sum  Inputs=+-
  Add2 : Sum
  Add3 : Sum
  Add4 : Sum  Inputs=+-
  Constant : Constant  SampleTime=Tsim
  Gain : Gain  Gain=1/Ld*Tsim
  Gain1 : Gain  Gain=Tsim/Ld
  Gain2 : Gain  Gain=K2*Tsim
  Gain3 : Gain  Gain=K1
  Gain5 : Gain  Gain=Tsim/Ld
  Product : Product
  Product1 : Product
  Sqrt : Sqrt  SaturateOnIntegerOverflow=on
  Step : Step  Time=3  Before=0.732  After=0.732+1.3  SampleTime=Tsim
  Subsystem : Subsystem
  Unit Delay1 : UnitDelay  SampleTime=-1  HasFrameUpgradeWarning=on
  Unit Delay2 : UnitDelay  SampleTime=-1  HasFrameUpgradeWarning=on
  Unit Delay3 : UnitDelay  SampleTime=-1  HasFrameUpgradeWarning=on
  Output : Outport
  wires:
  Gain2/1 -> Add3/1
  Add3/1 -> Unit Delay3/1
  Add/1 -> Unit Delay1/1
  Gain5/1 -> Add/1
  Product/1 -> Unit Delay2/1
  Subsystem/1(Out1) -> Gain2/1, Product/2
  Gain1/1 -> Add/2
  Add2/1 -> Output/1, Gain5/1  "Est_Ealpha"
  Product1/1 -> Add/3
  Gain3/1 -> Product/1
  Sqrt/1 -> Gain3/1
  U/1 -> Gain1/1
  I/1 -> Add1/2
  Add1/1 -> Subsystem/1(In1), Abs/1
  Abs/1 -> Sqrt/1
  Unit Delay1/1 -> Add1/1, Product1/2
  Unit Delay2/1 -> Add2/1
  Unit Delay3/1 -> Add3/2, Add2/2
  Add4/1 -> Product1/1
  Constant/1 -> Add4/1
  Step/1 -> Gain/1
  Gain/1 -> Add4/2

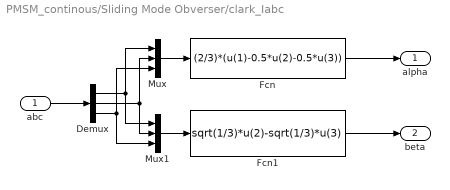
== system PMSM_continous/Sliding Mode Obverser/clark_Iabc ==
  abc : Inport
  Demux : Demux  Outputs=3
  Fcn : Fcn  Expr=(2/3)*(u(1)-0.5*u(2)-0.5*u(3))
  Fcn1 : Fcn  Expr=sqrt(1/3)*u(2)-sqrt(1/3)*u(3)
  Mux : Mux  Inputs=3
  Mux1 : Mux  Inputs=3
  alpha : Outport  VectorParamsAs1DForOutWhenUnconnected=off
  beta : Outport  Port=2  VectorParamsAs1DForOutWhenUnconnected=off
  wires:
  abc/1 -> Demux/1
  Fcn/1 -> alpha/1
  Demux/1 -> Mux1/1, Mux/1
  Demux/2 -> Mux1/2, Mux/2
  Mux/1 -> Fcn/1
  Demux/3 -> Mux1/3, Mux/3
  Fcn1/1 -> beta/1
  Mux1/1 -> Fcn1/1

== system PMSM_continous/Sliding Mode Obverser/clark_Iabc1 ==
  abc : Inport
  Demux : Demux  Outputs=3
  Fcn : Fcn  Expr=(2/3)*(u(1)-0.5*u(2)-0.5*u(3))
  Fcn1 : Fcn  Expr=sqrt(1/3)*u(2)-sqrt(1/3)*u(3)
  Mux : Mux  Inputs=3
  Mux1 : Mux  Inputs=3
  alpha : Outport  VectorParamsAs1DForOutWhenUnconnected=off
  beta : Outport  Port=2  VectorParamsAs1DForOutWhenUnconnected=off
  wires:
  abc/1 -> Demux/1
  Fcn/1 -> alpha/1
  Demux/1 -> Mux1/1, Mux/1
  Demux/2 -> Mux1/2, Mux/2
  Mux/1 -> Fcn/1
  Demux/3 -> Mux1/3, Mux/3
  Fcn1/1 -> beta/1
  Mux1/1 -> Fcn1/1

== system PMSM_continous/Sliding Mode Obverser/clark_Vabc ==
  abc : Inport
  Demux : Demux  Outputs=3
  Fcn : Fcn  Expr=(2/3)*(u(1)-0.5*u(2)-0.5*u(3))
  Fcn1 : Fcn  Expr=sqrt(1/3)*u(2)-sqrt(1/3)*u(3)
  Mux : Mux  Inputs=3
  Mux1 : Mux  Inputs=3
  alpha : Outport  VectorParamsAs1DForOutWhenUnconnected=off
  beta : Outport  Port=2  VectorParamsAs1DForOutWhenUnconnected=off
  wires:
  abc/1 -> Demux/1
  Fcn/1 -> alpha/1
  Demux/1 -> Mux1/1, Mux/1
  Demux/2 -> Mux1/2, Mux/2
  Mux/1 -> Fcn/1
  Demux/3 -> Mux1/3, Mux/3
  Fcn1/1 -> beta/1
  Mux1/1 -> Fcn1/1

== system PMSM_continous/Sliding Mode Obverser/clark_Vabc1 ==
  abc : Inport
  Demux : Demux  Outputs=3
  Fcn : Fcn  Expr=(2/3)*(u(1)-0.5*u(2)-0.5*u(3))
  Fcn1 : Fcn  Expr=sqrt(1/3)*u(2)-sqrt(1/3)*u(3)
  Mux : Mux  Inputs=3
  Mux1 : Mux  Inputs=3
  alpha : Outport  VectorParamsAs1DForOutWhenUnconnected=off
  beta : Outport  Port=2  VectorParamsAs1DForOutWhenUnconnected=off
  wires:
  abc/1 -> Demux/1
  Fcn/1 -> alpha/1
  Demux/1 -> Mux1/1, Mux/1
  Demux/2 -> Mux1/2, Mux/2
  Mux/1 -> Fcn/1
  Demux/3 -> Mux1/3, Mux/3
  Fcn1/1 -> beta/1
  Mux1/1 -> Fcn1/1

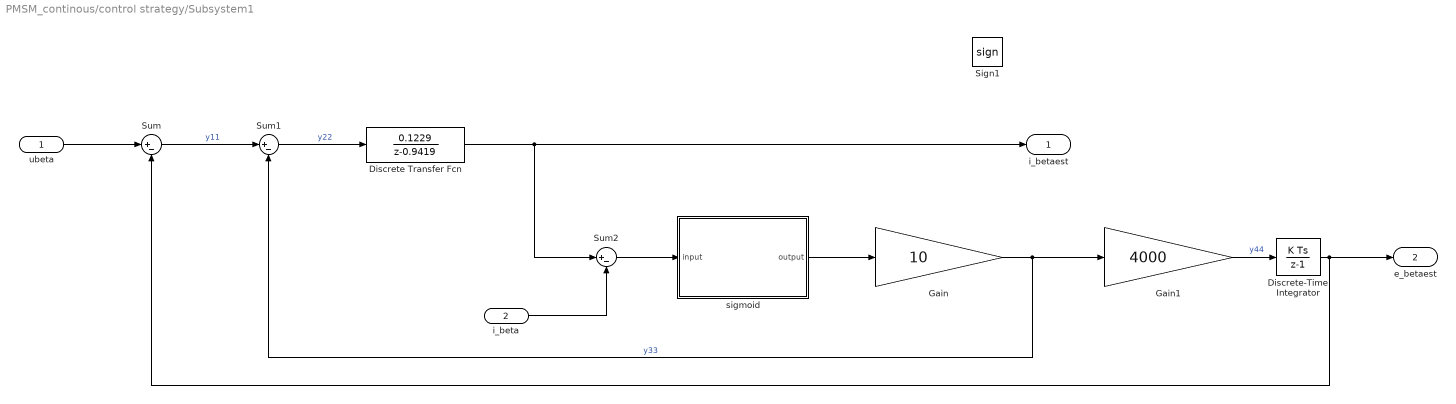
== system PMSM_continous/control strategy/Subsystem1 ==
  ubeta : Inport
  i_beta : Inport  Port=2
  Discrete Transfer Fcn : DiscreteTransferFcn  Numerator=[0.1229]  Denominator=[1 -0.9419]  SampleTime=Ts
  Discrete-Time Integrator : DiscreteIntegrator  SampleTime=Ts  UpperSaturationLimit=UpperLimit  LowerSaturationLimit=LowerLimit  ICPrevOutput=DiscIntNeverNeededParam  ICPrevScaledInput=DiscIntNeverNeededParam
  Gain : Gain  Gain=10
  Gain1 : Gain  Gain=4000
  Sign1 : Signum
  Sum : Sum  Inputs=|+-
  Sum1 : Sum  Inputs=|+-
  Sum2 : Sum  Inputs=|+-
  sigmoid : Subsystem
  i_betaest : Outport  VectorParamsAs1DForOutWhenUnconnected=off
  e_betaest : Outport  Port=2  VectorParamsAs1DForOutWhenUnconnected=off
  wires:
  Sum2/1 -> sigmoid/1(input)
  Gain/1 -> Gain1/1, Sum1/2  "y33"
  i_beta/1 -> Sum2/2
  Discrete Transfer Fcn/1 -> Sum2/1, i_betaest/1
  Sum/1 -> Sum1/1  "y11"
  ubeta/1 -> Sum/1
  Sum1/1 -> Discrete Transfer Fcn/1  "y22"
  Gain1/1 -> Discrete-Time Integrator/1  "y44"
  sigmoid/1(output) -> Gain/1
  Discrete-Time Integrator/1 -> e_betaest/1, Sum/2

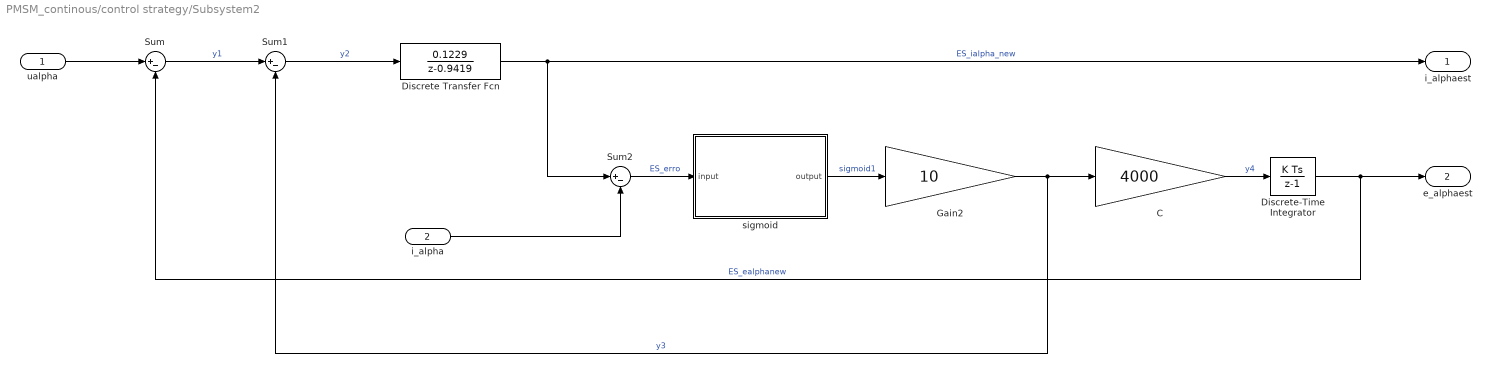
== system PMSM_continous/control strategy/Subsystem2 ==
  ualpha : Inport
  i_alpha : Inport  Port=2
  C : Gain  Gain=4000
  Discrete Transfer Fcn : DiscreteTransferFcn  Numerator=[0.1229]  Denominator=[1 -0.9419]  SampleTime=Ts
  Discrete-Time Integrator : DiscreteIntegrator  SampleTime=Ts  UpperSaturationLimit=UpperLimit  LowerSaturationLimit=LowerLimit  ICPrevOutput=DiscIntNeverNeededParam  ICPrevScaledInput=DiscIntNeverNeededParam
  Gain2 : Gain  Gain=10
  Sum : Sum  Inputs=|+-
  Sum1 : Sum  Inputs=|+-
  Sum2 : Sum  Inputs=|+-
  sigmoid : Subsystem
  i_alphaest : Outport  VectorParamsAs1DForOutWhenUnconnected=off
  e_alphaest : Outport  Port=2  VectorParamsAs1DForOutWhenUnconnected=off
  wires:
  C/1 -> Discrete-Time Integrator/1  "y4"
  Sum1/1 -> Discrete Transfer Fcn/1  "y2"
  ualpha/1 -> Sum/1
  sigmoid/1(output) -> Gain2/1  "sigmoid1"
  Sum/1 -> Sum1/1  "y1"
  Discrete Transfer Fcn/1 -> i_alphaest/1, Sum2/1  "ES_ialpha_new"
  i_alpha/1 -> Sum2/2
  Sum2/1 -> sigmoid/1(input)  "ES_erro"
  Gain2/1 -> C/1, Sum1/2  "y3"
  Discrete-Time Integrator/1 -> Sum/2, e_alphaest/1  "ES_ealphanew"

== system PMSM_continous/control strategy/clark ==
  iabc : Inport
  Demux : Demux  Outputs=3
  Fcn : Fcn  Expr=(2/3)*(u(1)-0.5*u(2)-0.5*u(3))
  Fcn1 : Fcn  Expr=sqrt(1/3)*u(2)-sqrt(1/3)*u(3)
  Mux : Mux  Inputs=3
  Mux1 : Mux  Inputs=3
  ialf : Outport  VectorParamsAs1DForOutWhenUnconnected=off
  ibate : Outport  Port=2  VectorParamsAs1DForOutWhenUnconnected=off
  wires:
  iabc/1 -> Demux/1
  Fcn/1 -> ialf/1
  Demux/1 -> Mux1/1, Mux/1
  Demux/2 -> Mux1/2, Mux/2
  Mux/1 -> Fcn/1
  Demux/3 -> Mux1/3, Mux/3
  Fcn1/1 -> ibate/1
  Mux1/1 -> Fcn1/1

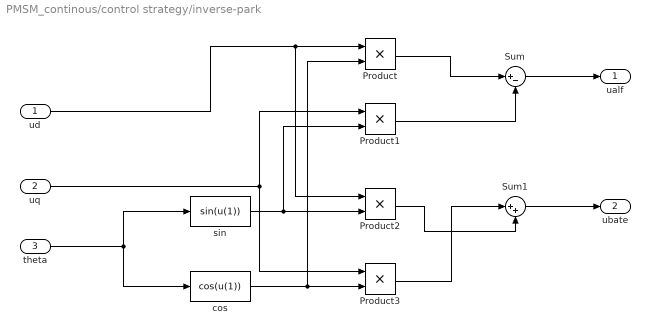
== system PMSM_continous/control strategy/inverse-park ==
  ud : Inport
  uq : Inport  Port=2
  theta : Inport  Port=3
  Product{,1..3} (4 alike) : Product
  Sum : Sum  Inputs=|+-
  Sum1 : Sum  Inputs=|++
  cos : Fcn  Expr=cos(u(1))
  sin : Fcn  Expr=sin(u(1))
  "ualf " : Outport  VectorParamsAs1DForOutWhenUnconnected=off
  ubate : Outport  Port=2  VectorParamsAs1DForOutWhenUnconnected=off
  wires:
  cos/1 -> Product3/2, Product/2
  sin/1 -> Product2/2, Product1/2
  Sum/1 -> "ualf "/1
  Product3/1 -> Sum1/1
  Product2/1 -> Sum1/2
  theta/1 -> cos/1, sin/1
  Product1/1 -> Sum/2
  Product/1 -> Sum/1
  Sum1/1 -> ubate/1
  uq/1 -> Product3/1, Product1/1
  ud/1 -> Product2/1, Product/1

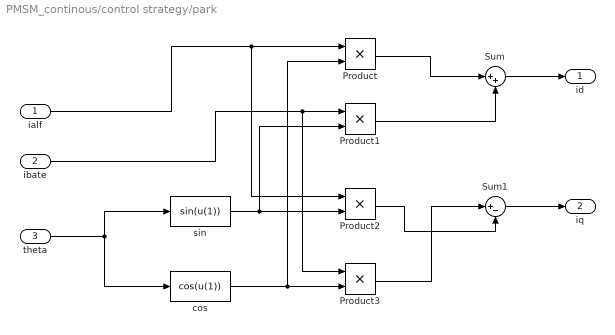
== system PMSM_continous/control strategy/park ==
  ialf : Inport
  ibate : Inport  Port=2
  theta : Inport  Port=3
  Product{,1..3} (4 alike) : Product
  Sum : Sum  Inputs=|++
  Sum1 : Sum  Inputs=|+-
  cos : Fcn  Expr=cos(u(1))
  sin : Fcn  Expr=sin(u(1))
  "id " : Outport  VectorParamsAs1DForOutWhenUnconnected=off
  iq : Outport  Port=2  VectorParamsAs1DForOutWhenUnconnected=off
  wires:
  Sum1/1 -> iq/1
  Product3/1 -> Sum1/1
  theta/1 -> cos/1, sin/1
  Sum/1 -> "id "/1
  Product2/1 -> Sum1/2
  ibate/1 -> Product3/1, Product1/1
  Product/1 -> Sum/1
  sin/1 -> Product2/2, Product1/2
  Product1/1 -> Sum/2
  ialf/1 -> Product2/1, Product/1
  cos/1 -> Product3/2, Product/2

== system PMSM_continous/Sliding Mode Obverser/Subsystem1/Subsystem ==
  In1 : Inport
  Add5 : Sum  Inputs=+-
  Constant1 : Constant  Value=0.5
  Gain4 : Gain  Gain=2
  Sigmoidal MF : fuzblock/Membership  Functions/Sigmoidal MF  a=sigmoid  c=0
      settings: SourceProductName=Fuzzy Logic Toolbox  SourceProductBaseCode=FL
  Out1 : Outport
  wires:
  Sigmoidal MF/1 -> Add5/1
  Add5/1 -> Gain4/1
  Constant1/1 -> Add5/2
  Gain4/1 -> Out1/1
  In1/1 -> Sigmoidal MF/1

== system PMSM_continous/Sliding Mode Obverser/Subsystem2/Subsystem ==
  In1 : Inport
  Add5 : Sum  Inputs=+-
  Constant1 : Constant  Value=0.5
  Gain4 : Gain  Gain=2
  Sigmoidal MF : fuzblock/Membership  Functions/Sigmoidal MF  a=sigmoid  c=0
      settings: SourceProductName=Fuzzy Logic Toolbox  SourceProductBaseCode=FL
  Out1 : Outport
  wires:
  Sigmoidal MF/1 -> Add5/1
  Add5/1 -> Gain4/1
  Constant1/1 -> Add5/2
  Gain4/1 -> Out1/1
  In1/1 -> Sigmoidal MF/1

== system PMSM_continous/control strategy/Subsystem1/sigmoid ==
  input : Inport
  Add3 : Sum  Inputs=+-
  Constant : Constant
  Gain1 : Gain  Gain=2
  Sigmoidal MF1 : fuzblock/Membership  Functions/Sigmoidal MF  a=siga  c=0
      settings: SourceProductName=Fuzzy Logic Toolbox  SourceProductBaseCode=FL
  output : Outport  VectorParamsAs1DForOutWhenUnconnected=off
  wires:
  Constant/1 -> Add3/2
  Gain1/1 -> Add3/1
  Add3/1 -> output/1
  input/1 -> Sigmoidal MF1/1
  Sigmoidal MF1/1 -> Gain1/1

== system PMSM_continous/control strategy/Subsystem2/sigmoid ==
  input : Inport
  Add3 : Sum  Inputs=+-
  Constant : Constant
  Gain1 : Gain  Gain=2
  Sigmoidal MF1 : fuzblock/Membership  Functions/Sigmoidal MF  a=siga  c=0
      settings: SourceProductName=Fuzzy Logic Toolbox  SourceProductBaseCode=FL
  output : Outport  VectorParamsAs1DForOutWhenUnconnected=off
  wires:
  Sigmoidal MF1/1 -> Gain1/1
  input/1 -> Sigmoidal MF1/1
  Add3/1 -> output/1
  Gain1/1 -> Add3/1
  Constant/1 -> Add3/2

== matlab function PMSM_continous/Sliding Mode Obverser/SMO ==
  settings: updateMethod=DISCRETE
  data: Valpha input; Vbeta input; Ialpha input; est_theta output; Ibeta input; frequency input; est_EMF output
function [est_theta,est_EMF] = smo_observer(Valpha,Vbeta,Ialpha,Ibeta,frequency)
%slide 影响高速时的稳定性，slide越大，位置的高频谐波越小
%E0是误差，暂时没有发现其与相位的影响，怀疑slide是不是要随着转速越来越大才可以

Rs = 0.735;
Ls = 10.24*1e-3;
Ts = 1/2000000;
Kslf = frequency*Ts*2;
slide = 0.1385*frequency*50;
% Kslf = 40;

E0 = 0.005;

persistent EstIalpha Ealpha Zalpha; 
persistent EstIbeta Ebeta Zbeta; 
if isempty(EstIalpha)
    EstIalpha = 0;
end
if isempty(Ealpha)
    Ealpha = 0;
end  
if isempty(Zalpha)
    Zalpha = 0;
end


if isempty(EstIbeta)
    EstIbeta = 0;
end
if isempty(Ebeta)
    Ebeta = 0;
end  
if isempty(Zbeta)
    Zbeta = 0;
end
  
    Fsmopos = exp(-Rs*Ts/Ls);
    Gsmopos = (1/Rs)*(1-Fsmopos);

%     Fsmopos = 1-Rs*Ts/Ls;
%     Gsmopos = Ts*Ls;
    
    EstIalpha = Fsmopos*EstIalpha + Gsmopos*(Valpha - Ealpha - Zalpha);
    EstIbeta  = Fsmopos*EstIbeta  + Gsmopos*(Vbeta - Ebeta  - Zbeta );
    
    IalphaError =(EstIalpha - Ialpha);
    IbetaError = (EstIbeta - Ibeta);    
%     if(IalphaError > E0)
%         IalphaError = 1;
%     elseif(IalphaError < -E0)
%         IalphaError = -1;
%     end
%     if(IbetaError > E0)
%         IbetaError = 1;
%     elseif(IbetaError < -E0)
%         IbetaError = -1;
%     end        


%     Zalpha = (2.0./(1+exp(-E0*IalphaError))-1)*slide;
%     Zbeta = (2.0./(1+exp(-E0*IbetaError))-1)*slide;

    Zalpha = sign(IalphaError)*slide;
    Zbeta  = sign(IbetaError )*slide;
    
    Ealpha =Kslf*Zalpha + (1-Kslf)*Ealpha;
    Ebeta  =Kslf*Zbeta  + (1-Kslf)*Ebeta;
    
    
    est_theta = mod(atan2((-Ealpha),Ebeta)+pi-atan(1/2),2*pi);
    
    est_EMF = [Ealpha,Ebeta];

end

== matlab function PMSM_continous/Sliding Mode Obverser/MATLAB Function1 ==
  data: Ualpha input; Est_EMF output; Ubeta input; Ialpha input; Ibeta input; est_theta output
function [Est_EMF,est_theta] = Est_EMF(Ualpha,Ubeta,Ialpha,Ibeta)


Rs = 0.735;
Ls = 10.24*1e-3;
Ts = 500e-9;
K1 = 2;
K2 = 2000;
Kslf = 150*Ts;

persistent Est_Ialpha Est_Ibeta;
if isempty(Est_Ialpha)
    Est_Ialpha = 0;
end
if isempty(Est_Ibeta)
    Est_Ibeta = 0;
end

persistent Ealpha Ebeta;
if isempty(Ealpha)
    Ealpha = 0;
end
if isempty(Ebeta)
    Ebeta = 0;
end

persistent Zalpha Zbeta;
if isempty(Zalpha)
    Zalpha = 0;
end
if isempty(Zbeta)
    Zbeta = 0;
end

persistent EMF_alpha EMF_beta;
if isempty(EMF_alpha)
    EMF_alpha = 0;
end
if isempty(EMF_beta)
    EMF_beta = 0;
end


Est_Ialpha = (1 - Rs/Ls*Ts)*Est_Ialpha + Ts/Ls*(Ualpha - Ealpha);
Est_Ibeta  = (1 - Rs/Ls*Ts)*Est_Ibeta  + Ts/Ls*(Ubeta  - Ebeta );

IalphaError = real(Est_Ialpha - Ialpha);
IbetaError  = real(Est_Ibeta  -  Ibeta) ;

sqrt_IalphaError = real(sqrt(abs(IalphaError)));
sqrt_IbetaError  = real(sqrt(abs(IbetaError )));

Zalpha = real(Zalpha) + Ts*K2*sign(IalphaError);
Zbeta  = real(Zbeta)  + Ts*K2*sign(IbetaError );

Ealpha = K1*(sqrt_IalphaError)*sign(IalphaError) + real(Zalpha);
Ebeta  = K1*(sqrt_IbetaError )*sign(IbetaError ) + real(Zbeta );

EMF_alpha = Kslf*Ealpha + (1-Kslf)*EMF_alpha;
EMF_beta  = Kslf*Ebeta  + (1-Kslf)*EMF_beta ;



Est_EMF = [real(Ealpha),real(Ebeta)];

est_theta = mod(atan2(real(-EMF_alpha),real(EMF_beta)),2*pi);

== matlab function PMSM_continous/Sliding Mode Obverser/MATLAB Function ==
  data: electric_theta input; est_speed output; flag input
function est_speed = speed_estimated(electric_theta,flag)

Ts = 1/20000;
P = 10;


persistent old_theta estimatedspeed;
if isempty(old_theta)
    old_theta = 0;
end
if isempty(estimatedspeed)
    estimatedspeed = 0;
end

temp = electric_theta - old_theta;


if(temp < -pi)
    temp = temp + 2*pi;
elseif(temp > pi)
    temp = temp - 2*pi;
end
if(flag >0)
    estimatedspeed = temp/Ts;
    old_theta = electric_theta;
    est_speed = estimatedspeed*30/pi/P;
else
    est_speed = 0;
end

== matlab function PMSM_continous/Measurement /MATLAB Function ==
  data: est_theta input; error output; real_theta input
function error = error(est_theta,real_theta)

error = est_theta - real_theta;
if(error > pi)
    error = error - 2*pi;
elseif(error <- pi)
	error = error + 2*pi;
end

if(error>2*pi||error<-2*pi)
    error = 0;
end

== matlab function PMSM_continous/Sliding Mode Obverser/MATLAB Function2 ==
  data: alpha input; Est_theta output; beta input; compansite input
function Est_theta = atan2(alpha,beta,compansite)
Est_theta = atan2(-alpha,beta);
if Est_theta<0
    Est_theta = pi - Est_theta;
end

== matlab function PMSM_continous/Sliding Mode Obverser/MATLAB Function3 ==
  data: est_theta input; error output; real_theta input
function error = error(est_theta,real_theta)

error = est_theta - real_theta;
if(error > pi)
    error = error - 2*pi;
elseif(error <- pi)
	error = error + 2*pi;
end

if(error>2*pi||error<-2*pi)
    error = 0;
end

== matlab function PMSM_continous/control strategy/MATLAB Function1 ==
  data: Ud input; Ud_out output; Uq input; Uq_out output
function [Ud_out,Uq_out] = Over_Modulation(Ud,Uq)

Us = (Ud^2+Uq^2)^0.5;
if(Us>sqrt(3)/3)
    Ud_out = Ud/Us*sqrt(3)/3;
    Uq_out = Uq/Us*sqrt(3)/3;
else
    Ud_out = Ud;
    Uq_out = Uq;
end
    
end

== matlab function PMSM_continous/control strategy/MATLAB Function ==
  data: u input; y output
function y = fcn(u)
if (u<0.84)
    u = 0.84;
end
y = u;

== matlab function PMSM_continous/Measurement /MATLAB Function1 ==
  data: theta input; Ealpha output; Ebeta output
function [Ealpha,Ebeta] = EMF(theta)
Ealpha = -sin(theta);
Ebeta = cos(theta);

end
